simulink model "Simulink_Test"  (R2024a)
settings: Solver=FixedStepAuto  StartTime=0.0  StopTime=10.0  RelTol=1e-3  EnableMultiTasking=on
libraries: stm32f4xxblockslib x2, stm32blockslib x2
settings Model: STM32="{\"DigitalPortWrite\":[{\"ID\":\"Simulink_Test:4\"},{\"ID\":\"Simulink_Test:5\"}],\"UARTWrite\":{\"ID\":\"Simulink_Test:15\"},\"UARTRead\":{\"ID\":\"Simulink_Test:12\"}}"  Creator=86173  LastModifiedBy=86173
settings OptimizationCC: EnhancedBackFolding=on  PassReuseOutputArgsAs=Individual arguments  ZeroExternalMemoryAtStartup=off  ZeroInternalMemoryAtStartup=off  MaxStackSize=64  OptimizeBlockOrder=speed  DifferentSizesBufferReuse=on  OptimizationCustomize=off  EfficientTunableParamExpr=on
settings DebuggingCC: ParameterTunabilityLossMsg=error
settings HardwareCC: ProdBitPerPointer=32  ProdBitPerSizeT=32  ProdBitPerPtrDiffT=32  ProdLargestAtomicInteger=Long  ProdLargestAtomicFloat=Double  ProdWordSize=32  ProdLongLongMode=on  ProdHWDeviceType=ARM Compatible->ARM Cortex-M
settings SFSimCC: MATLABDynamicMemAlloc=off
settings RTWCC: Description=Embedded Coder  SystemTargetFile=ert.tlc  HardwareBoard=STM32F4xx Based  TemplateMakefile=ert_default_tmf  Toolchain=GNU Tools for ARM Embedded Processors
settings CodeAppCC: ForceParamTrailComments=on  IgnoreCustomStorageClasses=off  OperatorAnnotations=on  SimulinkDataObjDesc=on  SFDataObjDesc=on  InsertBlockDesc=on
settings ERTTargetCC: TargetLangStandard=C99 (ISO)  CodeReplacementLibrary=ARM Cortex-M  ExtModeTransport=3  ExtModeStaticAlloc=on  ExtModeStaticAllocSize=2048  ExtModeMexFile=ext_xcp  ExtModeMexArgs=-port COM7 -b 115200 -t 20  ExtModeIntrfLevel=Level2 - Open

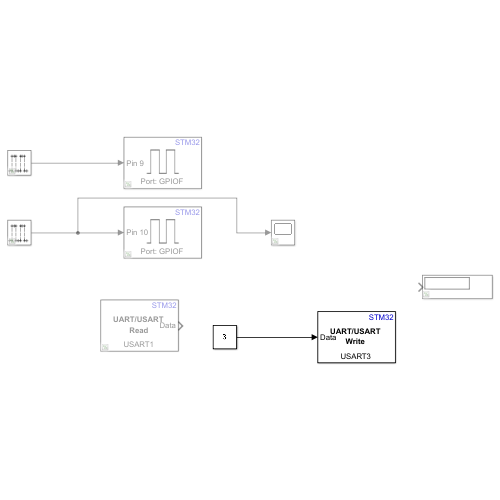
[thumbnail: Simulink's stored preview of the top-level diagram]
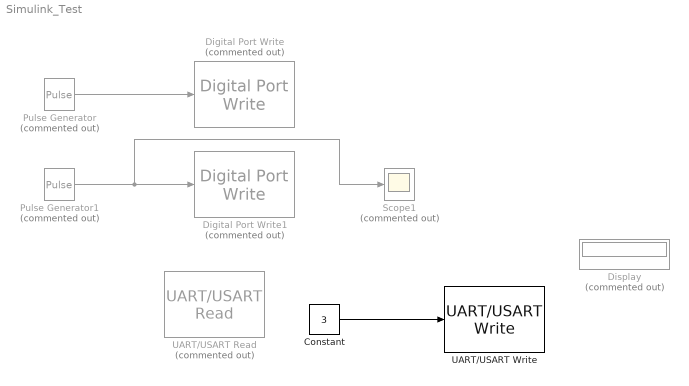
== system Simulink_Test ==
  Constant : Constant  Value=3  OutDataTypeStr=uint8
  Digital Port Write : stm32f4xxblockslib/Digital Port Write  Commented=on  PortName=GPIOF  PinNumber=9  ReadOperation=off  IOAsArray=off  EnableSimPort=off  hoistedMaskSrc=ECSoC/ECSimCodegen/Digital Port Write
  Digital Port Write1 : stm32f4xxblockslib/Digital Port Write  Commented=on  PortName=GPIOF  PinNumber=10  ReadOperation=off  IOAsArray=off  EnableSimPort=off  hoistedMaskSrc=ECSoC/ECSimCodegen/Digital Port Write
  Display : Display  Commented=on
  Pulse Generator : DiscretePulseGenerator  Commented=on  SampleTime=0.2
  Pulse Generator1 : DiscretePulseGenerator  Commented=on  SampleTime=0.2
  Scope1 : Scope  Commented=on
  UART/USART Read : stm32blockslib/UART//USART Read  Commented=on  UARTModule=USART1  DataType=uint8  DataLength=1  BlockingMode=off  BlockingTimeout=0.1  OutputLength=off  OutputStatus=off  SampleTime=-1
      settings: LibrarySourceBlock=stm32f4xxblockslib/UART//USART Read
  UART/USART Write : stm32blockslib/UART//USART Write  UARTModule=USART3  LengthOfDataToSend=off  BlockingMode=off  BlockingTimeout=0.1  OutputStatus=off
      settings: LibrarySourceBlock=stm32f4xxblockslib/UART//USART Write
  wires:
  Pulse Generator1/1 -> Scope1/1, Digital Port Write1/1
  Pulse Generator/1 -> Digital Port Write/1
  Constant/1 -> UART/USART Write/1
